simulink model "sltestMATLABBasedTestExample"  (R2025a)
settings: Solver=ode45  StartTime=0.0  StopTime=10.0  RelTol=1e-3  EnableMultiTasking=on
PostLoadFcn:
  | gain2_var = 2;
CloseFcn:
  | clear gain2_var;
Description:
  | sltestMATLABBasedTestExample model
  | This model is used to show how a MATLAB-Based Simulink test can be created
  | and then executed in the Test Manager.
settings Model: Creator=The MathWorks, Inc.  LastModifiedBy=vkayithi
settings SolverCC: AlgebraicLoopSolver=TrustRegion  MaxZcPerStep=1.0
settings DataIOCC: LimitDataPoints=on  SignalLogging=off  DSMLogging=off  SaveTime=off
settings OptimizationCC: LifeSpan=inf
settings DebuggingCC: UnconnectedInputMsg=warning  UnconnectedOutputMsg=warning  UnconnectedLineMsg=warning  SFUnexpectedBacktrackingDiag=warning  SFNoUnconditionalDefaultTransitionDiag=warning  SFExecutionAtInitializationDiag=none  ArithmeticOperatorsInVariantConditions=warning
settings HardwareCC: ProdBitPerPointer=32.0  ProdBitPerSizeT=32.0  ProdBitPerPtrDiffT=32.0  ProdLargestAtomicFloat=None  ProdIntDivRoundTo=Undefined  ProdEndianess=Unspecified  ProdWordSize=32.0  ProdHWDeviceType=32-bit Generic
settings ModelReferenceCC: EnableRefExpFcnMdlSchedulingChecks=on  PropagateSignalLabelsOutOfModel=off
settings SFSimCC: SimUseLocalCustomCode=off  CustomCodeUndefinedFunction=UseInterfaceOnly
settings RTWCC: RTWUseLocalCustomCode=off  GPUComputeCapability=3.5  DLArmComputeVersion=19.05
settings CodeAppCC: StateflowObjectComments=on
settings GRTTargetCC: TargetLangStandard=C89/C90 (ANSI)
settings ConfigComp: CovMetricSettings=dw  CovSaveCumulativeToWorkspaceVar=on  CovSaveSingleToWorkspaceVar=on  CovExternalEMLEnable=off  CovSFcnEnable=off

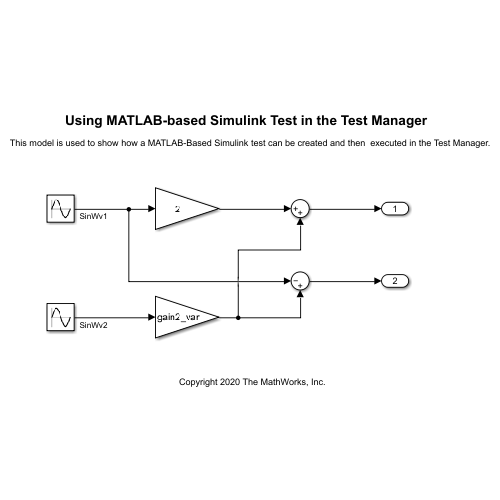
[thumbnail: Simulink's stored preview of the top-level diagram]
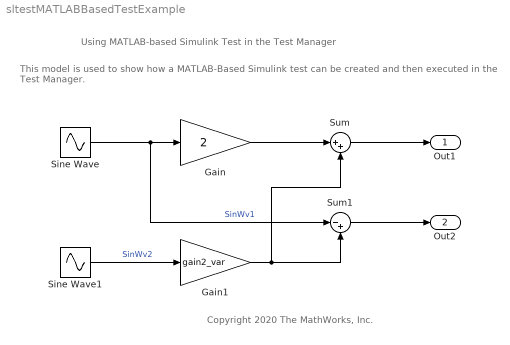
== system sltestMATLABBasedTestExample ==
  note: This model is used to show how a MATLAB-Based Simulink test can be created and then executed in the Test Manager.
  note: Using MATLAB-based Simulink Test in the Test Manager
  note: Copyright 2020 The MathWorks, Inc.
  Gain : Gain  Gain=2
  Gain1 : Gain  Gain=gain2_var
  Sine Wave : Sin  SampleTime=0
  Sine Wave1 : Sin  Phase=pi  SampleTime=0
  Sum : Sum  Inputs=|++
  Sum1 : Sum  Inputs=|-+
  Out1 : Outport
  Out2 : Outport  Port=2
  wires:
  Sine Wave/1 -> Gain/1, Sum1/1  "SinWv1"
  Gain/1 -> Sum/1
  Sum/1 -> Out1/1
  Sine Wave1/1 -> Gain1/1  "SinWv2"
  Sum1/1 -> Out2/1
  Gain1/1 -> Sum/2, Sum1/2
